simulink model "AC_PlugInCharging"  (R2023b)
settings: Solver=FixedStepAuto  StartTime=0.0  StopTime=282  FixedStep=0.001  RelTol=1e-3
settings Model: Creator=mcmas  LastModifiedBy=OWNER

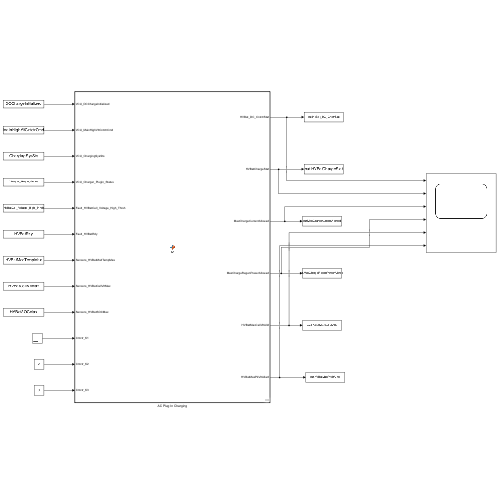
[thumbnail: Simulink's stored preview of the top-level diagram]
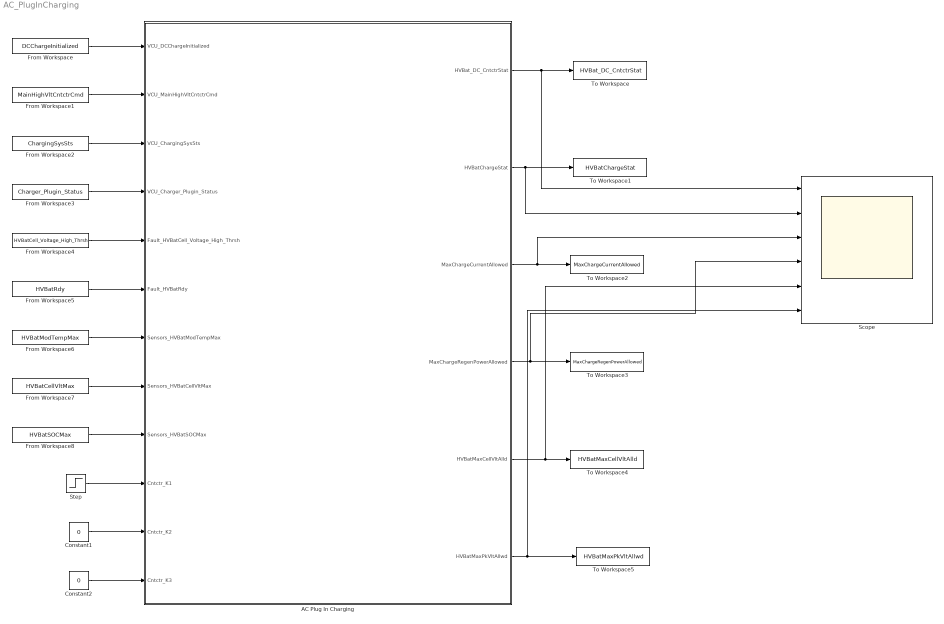
== system AC_PlugInCharging ==
  AC Plug In Charging : MATLAB Function  TreatAsAtomicUnit=on
  Constant1 : Constant  Value=0
  Constant2 : Constant  Value=0
  From Workspace : FromWorkspace  VariableName=DCChargeInitialized
  From Workspace1 : FromWorkspace  VariableName=MainHighVltCntctrCmd
  From Workspace2 : FromWorkspace  VariableName=ChargingSysSts
  From Workspace3 : FromWorkspace  VariableName=Charger_Plugin_Status
  From Workspace4 : FromWorkspace  VariableName=HVBatCell_Voltage_High_Thrsh
  From Workspace5 : FromWorkspace  VariableName=HVBatRdy
  From Workspace6 : FromWorkspace  VariableName=HVBatModTempMax
  From Workspace7 : FromWorkspace  VariableName=HVBatCellVltMax
  From Workspace8 : FromWorkspace  VariableName=HVBatSOCMax
  Scope : Scope  NumInputPorts=6
  Step : Step  Time=30  SampleTime=0
  To Workspace : ToWorkspace  VariableName=HVBat_DC_CntctrStat  SampleTime=-1
  To Workspace1 : ToWorkspace  VariableName=HVBatChargeStat  SampleTime=-1
  To Workspace2 : ToWorkspace  VariableName=MaxChargeCurrentAllowed  SampleTime=-1
  To Workspace3 : ToWorkspace  VariableName=MaxChargeRegenPowerAllowed  SampleTime=-1
  To Workspace4 : ToWorkspace  VariableName=HVBatMaxCellVltAlld  SampleTime=-1
  To Workspace5 : ToWorkspace  VariableName=HVBatMaxPkVltAllwd  SampleTime=-1
  wires:
  From Workspace/1 -> AC Plug In Charging/1(VCU_DCChargeInitialized)
  From Workspace1/1 -> AC Plug In Charging/2(VCU_MainHighVltCntctrCmd)
  From Workspace2/1 -> AC Plug In Charging/3(VCU_ChargingSysSts)
  From Workspace3/1 -> AC Plug In Charging/4(VCU_Charger_Plugin_Status)
  From Workspace4/1 -> AC Plug In Charging/5(Fault_HVBatCell_Voltage_High_Thrsh)
  From Workspace5/1 -> AC Plug In Charging/6(Fault_HVBatRdy)
  From Workspace6/1 -> AC Plug In Charging/7(Sensors_HVBatModTempMax)
  From Workspace7/1 -> AC Plug In Charging/8(Sensors_HVBatCellVltMax)
  From Workspace8/1 -> AC Plug In Charging/9(Sensors_HVBatSOCMax)
  Step/1 -> AC Plug In Charging/10(Cntctr_K1)
  Constant1/1 -> AC Plug In Charging/11(Cntctr_K2)
  Constant2/1 -> AC Plug In Charging/12(Cntctr_K3)
  AC Plug In Charging/1(HVBat_DC_CntctrStat) -> To Workspace/1, Scope/1
  AC Plug In Charging/2(HVBatChargeStat) -> To Workspace1/1, Scope/2
  AC Plug In Charging/3(MaxChargeCurrentAllowed) -> To Workspace2/1, Scope/3
  AC Plug In Charging/4(MaxChargeRegenPowerAllowed) -> To Workspace3/1, Scope/4
  AC Plug In Charging/5(HVBatMaxCellVltAlld) -> To Workspace4/1, Scope/5
  AC Plug In Charging/6(HVBatMaxPkVltAllwd) -> To Workspace5/1, Scope/6

== matlab function AC_PlugInCharging/AC Plug In Charging ==
  settings: updateMethod=DISCRETE
  data: HVBat_DC_CntctrStat output; VCU_DCChargeInitialized input; VCU_MainHighVltCntctrCmd input; VCU_ChargingSysSts input; VCU_Charger_Plugin_Status input; Fault_HVBatCell_Voltage_High_Thrsh input; Fault_HVBatRdy input; Sensors_HVBatModTempMax input; Sensors_HVBatCellVltMax input; Sensors_HVBatSOCMax input; Cntctr_K1 input; Cntctr_K2 input; Cntctr_K3 input; HVBatChargeStat output; MaxChargeCurrentAllowed output; MaxChargeRegenPowerAllowed output; HVBatMaxCellVltAlld output; HVBatMaxPkVltAllwd output
function [HVBat_DC_CntctrStat, HVBatChargeStat, MaxChargeCurrentAllowed, MaxChargeRegenPowerAllowed, HVBatMaxCellVltAlld, HVBatMaxPkVltAllwd] = ac( ...
    VCU_DCChargeInitialized, VCU_MainHighVltCntctrCmd, VCU_ChargingSysSts, VCU_Charger_Plugin_Status, ...
    Fault_HVBatCell_Voltage_High_Thrsh, Fault_HVBatRdy, ...
    Sensors_HVBatModTempMax, Sensors_HVBatCellVltMax, Sensors_HVBatSOCMax, Cntctr_K1, Cntctr_K2, Cntctr_K3)

% ===========================
%% INPUTS
% Time - Current time (s)
% VCU_MainHighVltCntctrCmd - VCU command for main contactor (0/1/2/3/7)
% Cntctr_K3,Cntctr_K2,Cntctr_K1 - Physical contactor feedbacks (1=closed, 0=open)
% Fault_HVBatRdy - Fault flag (0=Fault, 1=Ok)
% VCU_ChargingSysSts - 0=Not Charging,1=Charging,2=Interrupted,3=Complete
% VCU_Charger_Plugin_Status - 0=Unplugged, 1=Plugged
% Fault_HVBatCell_Voltage_High_Thrsh - Max allowable cell voltage (V)
% Sensors_HVBatModTempMax, Sensors_HVBatCellVltMax, Sensors_HVBatSOCMax - vectors
% VDC - DC bus voltage (V)
% HVBatMaxPkVltAllwd 
% HVBatMaxCellVltAlld

%% OUTPUTS
% HVBat_DC_CntctrStat - 0=Open, 1=Closed, 2=Faulted
% HVBatChargeStat     - 0=Not Ready, 1=Ready, 2=Charging, 3=Fault, 6=Complete
% MaxChargeCurrentAllowed - Allowed charging current (A)
% P_charge            - Estimated DC charging power (W)

%% --- Lookup Table for Max Charge Current [SOC vs Temp] ---
SOC = [0 5 10 15 20 25 30 35 40 45 50 55 60 65 70 75 80 85 90 95 100]; % 19 + 2 points
Temp = [-25 -20 -10 0 5 10 20 25 35 40 50]; % 11 points

ACChgCurrentProfile = [ ...
  0.05 0.05 0.05 0.05 0.05 0.05 0.05 0.05 0.05 0.05 0.05 0.05 0.05 0.02 0.02 0.01 0.01 0.01 0.01 0.01 0.00; ...
  0.06 0.06 0.06 0.06 0.06 0.06 0.06 0.06 0.06 0.06 0.06 0.06 0.06 0.02 0.02 0.02 0.02 0.01 0.01 0.01 0.00; ...
  0.45 0.45 0.45 0.45 0.45 0.15 0.15 0.15 0.15 0.09 0.09 0.09 0.09 0.03 0.03 0.03 0.03 0.02 0.02 0.02 0.00; ...
  0.70 0.70 0.70 0.70 0.70 0.70 0.70 0.70 0.70 0.50 0.50 0.50 0.50 0.25 0.25 0.25 0.25 0.10 0.10 0.09 0.00; ...
  0.85 0.85 0.85 0.85 0.85 0.85 0.85 0.85 0.85 0.75 0.75 0.75 0.75 0.63 0.63 0.58 0.44 0.35 0.24 0.12 0.00; ...
  0.88 0.88 0.88 0.88 0.88 0.88 0.88 0.88 0.88 0.88 0.88 0.88 0.88 0.88 0.88 0.68 0.59 0.35 0.24 0.12 0.00; ...
  0.88 0.88 0.88 0.88 0.88 0.88 0.88 0.88 0.88 0.88 0.88 0.88 0.88 0.88 0.88 0.88 0.74 0.59 0.44 0.29 0.00; ...
  0.88 0.88 0.88 0.88 0.88 0.88 0.88 0.88 0.88 0.88 0.88 0.88 0.88 0.88 0.88 0.88 0.88 0.74 0.59 0.44 0.00; ...
  0.88 0.88 0.88 0.88 0.88 0.88 0.88 0.88 0.88 0.88 0.88 0.88 0.88 0.88 0.88 0.88 0.88 0.74 0.65 0.59 0.00; ...
  0.88 0.88 0.88 0.88 0.88 0.88 0.88 0.88 0.88 0.88 0.88 0.88 0.88 0.88 0.88 0.88 0.88 0.76 0.74 0.60 0.00; ...
  0.88 0.88 0.88 0.88 0.88 0.88 0.88 0.88 0.88 0.88 0.88 0.88 0.88 0.88 0.88 0.88 0.88 0.60 0.60 0.48 0.00 ...
];

%% --- Calibrations ---
persistent Ke_t_DCFC_CntctrOpn Ke_T_HighChrgTempThresholdIn Ke_T_LowChrgTempThresholdIn ...
           Ke_U_ChargeCompletionVlt ...
           ParallelCellNum Ke_t_ChargeCompletionHold HVBatChargeTimer ...
           chargeCompleteFlag overTempFlag
if isempty(Ke_t_DCFC_CntctrOpn)
    Ke_t_DCFC_CntctrOpn = 1500;     % milliseconds      
    Ke_T_HighChrgTempThresholdIn = 50;   
    Ke_T_LowChrgTempThresholdIn  = -25;  
    Ke_U_ChargeCompletionVlt = 4.14;     
    ParallelCellNum = 34;
    Ke_t_ChargeCompletionHold = 300;     % milliseconds
    HVBatChargeTimer = 0;
    chargeCompleteFlag = false;
    overTempFlag = false;
end


persistent Ke_RegenVltMargin Ke_P_MaxChargeRegen
if isempty(Ke_RegenVltMargin)
    Ke_RegenVltMargin   = 0.05;   % [V] margin below Fault_HVBatCell_Voltage_High_Thrsh
    Ke_P_MaxChargeRegen = 11000;  % [W] max allowed regen during charge
end

%% --- Persistent states ---
persistent HVBatChargeStat_Aux MaxChargeCurrentAllowed_Aux MaxChargeRegenPowerAllowed_Aux
if isempty(HVBatChargeStat_Aux)
    HVBatChargeStat_Aux = 0;
    MaxChargeCurrentAllowed_Aux = 0;
    MaxChargeRegenPowerAllowed_Aux = 0;
end

%% Default outputs 
HVBatChargeStat = HVBatChargeStat_Aux;
MaxChargeCurrentAllowed = MaxChargeCurrentAllowed_Aux;
MaxChargeRegenPowerAllowed = MaxChargeRegenPowerAllowed_Aux;

%% --- AC Plug-in readiness
ready_cond = (VCU_DCChargeInitialized == 0) && (VCU_Charger_Plugin_Status == 1) && ~chargeCompleteFlag && ~overTempFlag;
main_contactor_ok = (VCU_MainHighVltCntctrCmd == 1) && (Cntctr_K1 == 1) && (Cntctr_K2 == 0) && (Cntctr_K3 == 0);

if ready_cond
    if main_contactor_ok && Fault_HVBatRdy == 1
        HVBatChargeStat_Aux = 1; % Ready
    else
        HVBatChargeStat_Aux = 0; % Not Ready
    end
elseif VCU_Charger_Plugin_Status == 1 && chargeCompleteFlag
    HVBatChargeStat_Aux = 6; % Complete
else
    HVBatChargeStat_Aux = 0; % Not Ready
end
MaxChargeCurrentAllowed_Aux = 0;
MaxChargeRegenPowerAllowed_Aux = 0;

%% Charging logic
Temp_actual = Sensors_HVBatModTempMax;
SOC_actual  = Sensors_HVBatSOCMax;
Vmax = Sensors_HVBatCellVltMax;

handshake_ok = (HVBatChargeStat_Aux == 1 && VCU_ChargingSysSts == 1);
if handshake_ok
    HVBatChargeStat_Aux = 2; % charge allow current
    if ~chargeCompleteFlag && ~overTempFlag && Temp_actual < Ke_T_HighChrgTempThresholdIn && Temp_actual > Ke_T_LowChrgTempThresholdIn && Vmax < Ke_U_ChargeCompletionVlt
        MaxChargeCurrentAllowed_Aux = ParallelCellNum * interp2(SOC, Temp, ACChgCurrentProfile, SOC_actual, Temp_actual);
    end
end

%% --- Charge Completion
if (HVBatChargeStat_Aux == 2) && ...
       (VCU_ChargingSysSts == 1 || VCU_ChargingSysSts == 3) && ...
       (Vmax >= Ke_U_ChargeCompletionVlt) && ...
       (~chargeCompleteFlag) && ...
       (~overTempFlag)
    if HVBatChargeTimer < 0
        HVBatChargeTimer = 0;
    end
    HVBatChargeTimer = HVBatChargeTimer + 1;
    if HVBatChargeTimer >= Ke_t_ChargeCompletionHold
        HVBatChargeStat_Aux = 6;
        MaxChargeCurrentAllowed_Aux = 0;
        MaxChargeRegenPowerAllowed_Aux = 0;
        chargeCompleteFlag = true;
    end
else
    HVBatChargeTimer = -1;
end

%% --- Overtemperature
if Temp_actual >= Ke_T_HighChrgTempThresholdIn || Temp_actual <= Ke_T_LowChrgTempThresholdIn
    HVBatChargeStat_Aux = 3;
    MaxChargeCurrentAllowed_Aux = 0;
    MaxChargeRegenPowerAllowed_Aux = 0;
    overTempFlag = true;
elseif overTempFlag && Temp_actual <= (Ke_T_HighChrgTempThresholdIn - 5) && Temp_actual >= (Ke_T_LowChrgTempThresholdIn + 5)
    overTempFlag = false;
end

%% --- Regen Power Limit
if VCU_ChargingSysSts == 1
    if Vmax >= Fault_HVBatCell_Voltage_High_Thrsh
        % No regen allowed at or above max allowable cell voltage
        MaxChargeCurrentAllowed_Aux = 0;
        MaxChargeRegenPowerAllowed_Aux = 0;
    
    elseif Vmax >= (Fault_HVBatCell_Voltage_High_Thrsh - Ke_RegenVltMargin)
        % Linearly reduce regen as voltage approaches limit
        scale = (Fault_HVBatCell_Voltage_High_Thrsh - Vmax) / Ke_RegenVltMargin;
        MaxChargeRegenPowerAllowed_Aux = max(0, scale * Ke_P_MaxChargeRegen);
    
    else
        % Full regen allowed (charge-mode limited)
        MaxChargeRegenPowerAllowed_Aux = Ke_P_MaxChargeRegen;
    end
end

% Fault handling
if (VCU_ChargingSysSts == 1 && Fault_HVBatRdy == 0)
    HVBatChargeStat_Aux = 3;
    MaxChargeCurrentAllowed_Aux = 0;
    MaxChargeRegenPowerAllowed_Aux = 0;
end

%% Overvoltage handling
if Vmax > Fault_HVBatCell_Voltage_High_Thrsh
    HVBatChargeStat_Aux = 3;
    MaxChargeCurrentAllowed_Aux = 0;
    MaxChargeRegenPowerAllowed_Aux = 0;
end

%% Reset completion flag ONLY when unplugged
if VCU_Charger_Plugin_Status == 0
    chargeCompleteFlag = false;
end

%% Outputs
HVBatChargeStat = HVBatChargeStat_Aux;
MaxChargeCurrentAllowed = MaxChargeCurrentAllowed_Aux;
MaxChargeRegenPowerAllowed = MaxChargeRegenPowerAllowed_Aux;
if isnan(MaxChargeCurrentAllowed), MaxChargeCurrentAllowed = 0; end
if isnan(MaxChargeRegenPowerAllowed), MaxChargeRegenPowerAllowed = 0; end

%% --- Step 3: Update Max Voltages
HVBatMaxCellVltAlld = Fault_HVBatCell_Voltage_High_Thrsh;
HVBatMaxPkVltAllwd = Fault_HVBatCell_Voltage_High_Thrsh * 105; % example for 105 series cells

%% DC Contactor state will always be open
HVBat_DC_CntctrStat = 0;

end
